simulink model "modal_control_siso_open_loop_system"  (R2020b)
settings: Solver=VariableStepAuto  StartTime=0.0  StopTime=200  RelTol=1e-3
values from neighbouring files (symbols this model uses):
  COUPLING_COEFFICIENT = 0.5736    [Workshop_MATLAB.m]
  FLEXIBLE_MODE_DAMPING_RATIO = 0.00495    [Workshop_MATLAB.m]
  FLEXIBLE_MODE_FREQUENCY = 2.6268    [Workshop_MATLAB.m]
  INITIAL_CONDITION_ON_STATE = 0.0001    [Workshop_MATLAB.m]
  REACTION_WHEEL_DYNAMICS_DENOMINATOR = [1 2.400 0.763]    [Workshop_MATLAB.m]
  REACTION_WHEEL_DYNAMICS_NUMERATOR = REACTION_WHEEL_INERTIA*[1.214 0.763 0]    [Workshop_MATLAB.m]
  REACTION_WHEEL_INERTIA = 0.0004    [Workshop_MATLAB.m]
  SATELLITE_INERTIA = 31.38    [Workshop_MATLAB.m]
settings Model: Creator=WLCG  LastModifiedBy=WLCG

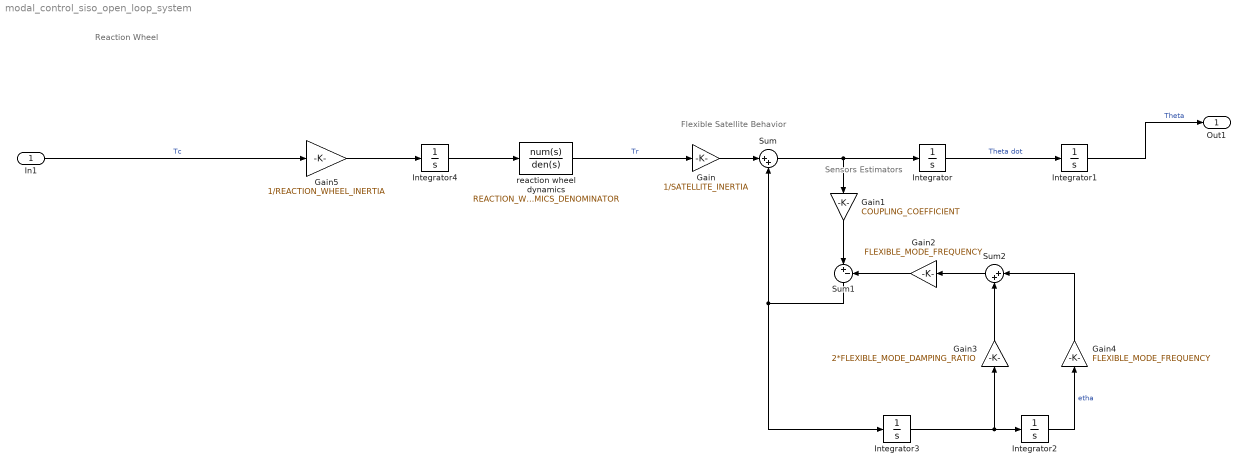
== system modal_control_siso_open_loop_system ==
  note: Reaction Wheel
  note: Sensors Estimators
  note: Flexible Satellite Behavior
  In1 : Inport
  Gain : Gain  Gain=1/SATELLITE_INERTIA
  Gain1 : Gain  Gain=COUPLING_COEFFICIENT
  Gain2 : Gain  Gain=FLEXIBLE_MODE_FREQUENCY
  Gain3 : Gain  Gain=2*FLEXIBLE_MODE_DAMPING_RATIO
  Gain4 : Gain  Gain=FLEXIBLE_MODE_FREQUENCY
  Gain5 : Gain  Gain=1/REACTION_WHEEL_INERTIA
  Integrator{,1,3..4} (4 alike) : Integrator
  Integrator2 : Integrator  InitialCondition=INITIAL_CONDITION_ON_STATE
  Sum : Sum  Inputs=|++
  Sum1 : Sum  Inputs=|+-
  Sum2 : Sum  Inputs=|++
  reaction wheel dynamics : TransferFcn  Numerator=REACTION_WHEEL_DYNAMICS_NUMERATOR  Denominator=REACTION_WHEEL_DYNAMICS_DENOMINATOR
  Out1 : Outport  SignalName=Theta
  wires:
  Sum2/1 -> Gain2/1
  Gain5/1 -> Integrator4/1
  Integrator4/1 -> reaction wheel dynamics/1
  In1/1 -> Gain5/1  "Tc"
  reaction wheel dynamics/1 -> Gain/1  "Tr"
  Integrator1/1 -> Out1/1  "Theta"
  Gain/1 -> Sum/1
  Gain3/1 -> Sum2/2
  Gain1/1 -> Sum1/1
  Sum1/1 -> Sum/2, Integrator3/1
  Integrator3/1 -> Integrator2/1, Gain3/1
  Gain4/1 -> Sum2/1
  Integrator2/1 -> Gain4/1  "etha"
  Gain2/1 -> Sum1/2
  Integrator/1 -> Integrator1/1  "Theta dot"
  Sum/1 -> Gain1/1, Integrator/1
